simulink model "PLANT"  (R2020b)
settings: Solver=VariableStepAuto  StartTime=0.0  StopTime=10  RelTol=1e-3
undefined symbols (not defined in the file): b, m
settings Model: Creator=priyaD  LastModifiedBy=priyaD
settings DataIOCC: SaveOutput=off  SaveTime=off

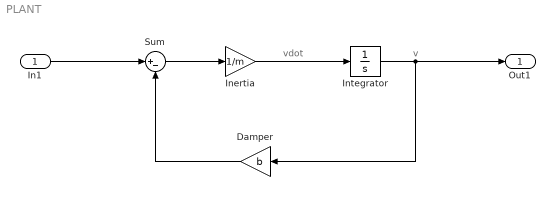
== system PLANT ==
  note: vdot
  note: v
  In1 : Inport  OutDataTypeStr=double  PortDimensions=1  SampleTime=0
  Damper : Gain  Gain=b
  Inertia : Gain  Gain=1/m
  Integrator : Integrator
  Sum : Sum  Inputs=|+-
  Out1 : Outport  OutDataTypeStr=double  PortDimensions=1  SampleTime=0
  wires:
  Sum/1 -> Inertia/1
  Damper/1 -> Sum/2
  In1/1 -> Sum/1
  Integrator/1 -> Damper/1, Out1/1
  Inertia/1 -> Integrator/1
